simulink model "LineEquation"  (R2021a)
settings: Solver=VariableStepAuto  StartTime=0.0  StopTime=10.0  RelTol=1e-3
settings Model: Creator=lenovo  LastModifiedBy=lenovo

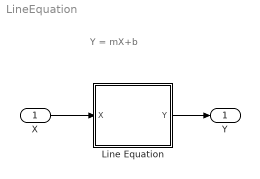
== system LineEquation ==
  note: Y = mX+b
  X : Inport
  Line Equation : Subsystem  mask{m=0, b=0}
      mask prompts: m "Slope"; b "Intersection"
      mask DialogControl DescGroupVar Prompt: Line Equation
  Y : Outport
  wires:
  X/1 -> Line Equation/1(X)
  Line Equation/1(Y) -> Y/1

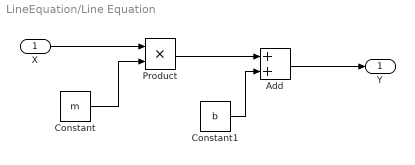
== system LineEquation/Line Equation ==
  X : Inport
  Add : Sum
  Constant : Constant  Value=m
  Constant1 : Constant  Value=b
  Product : Product
  Y : Outport
  wires:
  Add/1 -> Y/1
  Constant/1 -> Product/2
  Constant1/1 -> Add/2
  Product/1 -> Add/1
  X/1 -> Product/1
